simulink model "fu01"  (Simulink 5.0)
settings: Solver=ode45  StartTime=0.0  StopTime=inf  MaxStep=1/5000  MinStep=1/100000000  RelTol=1e-6
libraries: commcontsrc2 x1
settings Model: LastModifiedBy=efst

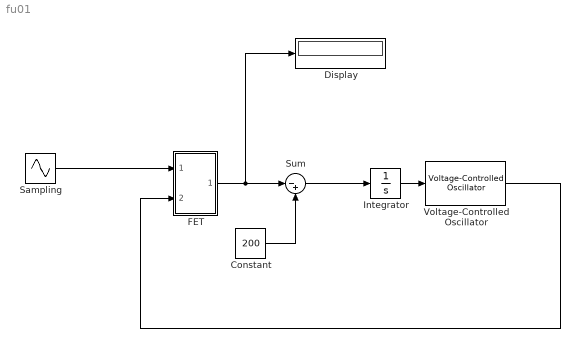
== system fu01 ==
  Constant : Constant  Value=200
  Display : Display
  FET : Subsystem
  Integrator : Integrator
  Sampling : Sin  Frequency=2*pi*1000  SampleTime=0
  Sum : Sum  Inputs=|-+  SaturateOnIntegerOverflow=on
  Voltage-Controlled Oscillator : commcontsrc2/Voltage-Controlled Oscillator  Ac=1  Fc=10  Kc=100  Ph=0
  wires:
  FET/1(Out1) -> Display/1, Sum/1
  Sampling/1 -> FET/1(In1)
  Integrator/1 -> Voltage-Controlled Oscillator/1
  Voltage-Controlled Oscillator/1 -> FET/2(In2)
  Sum/1 -> Integrator/1
  Constant/1 -> Sum/2

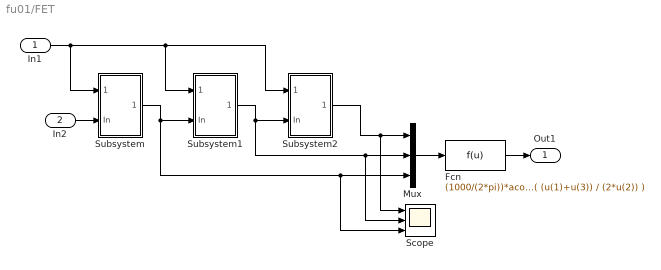
== system fu01/FET ==
  In1 : Inport
  In2 : Inport  Port=2
  Fcn : Fcn  Expr=(1000/(2*pi))*acos( (u(1)+u(3)) / (2*u(2)) )
  Mux : Mux  Inputs=3
  Scope : Scope  NumInputPorts=3
      settings: TimeRange=0.02  YMin=-1~-1~-1  YMax=1~1~1
  Subsystem : Subsystem
  Subsystem1 : Subsystem
  Subsystem2 : Subsystem
  Out1 : Outport
  wires:
  In1/1 -> Subsystem/1(Sample), Subsystem1/1(Sample), Subsystem2/1(Sample)
  Mux/1 -> Fcn/1
  Subsystem2/1(Out) -> Mux/1, Scope/1
  Subsystem1/1(Out) -> Subsystem2/2(In), Mux/2, Scope/2
  Subsystem/1(Out) -> Subsystem1/2(In), Mux/3, Scope/3
  In2/1 -> Subsystem/2(In)
  Fcn/1 -> Out1/1

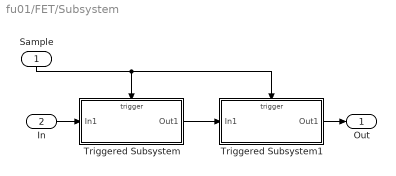
== system fu01/FET/Subsystem ==
  Sample : Inport  Orientation=down
  In : Inport  Port=2
  Triggered Subsystem : Subsystem  TreatAsAtomicUnit=on
  Triggered Subsystem1 : Subsystem  TreatAsAtomicUnit=on
  Out : Outport
  wires:
  Triggered Subsystem/1(Out1) -> Triggered Subsystem1/1(In1)
  Sample/1 -> Triggered Subsystem1/Trigger, Triggered Subsystem/Trigger
  In/1 -> Triggered Subsystem/1(In1)
  Triggered Subsystem1/1(Out1) -> Out/1

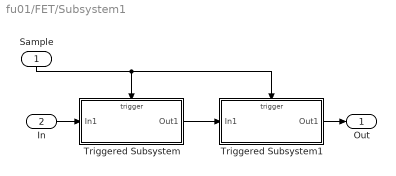
== system fu01/FET/Subsystem1 ==
  Sample : Inport  Orientation=down
  In : Inport  Port=2
  Triggered Subsystem : Subsystem  TreatAsAtomicUnit=on
  Triggered Subsystem1 : Subsystem  TreatAsAtomicUnit=on
  Out : Outport
  wires:
  Triggered Subsystem1/1(Out1) -> Out/1
  In/1 -> Triggered Subsystem/1(In1)
  Sample/1 -> Triggered Subsystem/Trigger, Triggered Subsystem1/Trigger
  Triggered Subsystem/1(Out1) -> Triggered Subsystem1/1(In1)

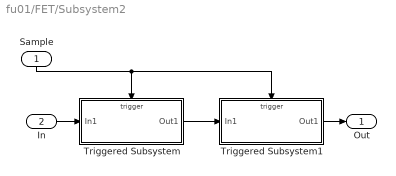
== system fu01/FET/Subsystem2 ==
  Sample : Inport  Orientation=down
  In : Inport  Port=2
  Triggered Subsystem : Subsystem  TreatAsAtomicUnit=on
  Triggered Subsystem1 : Subsystem  TreatAsAtomicUnit=on
  Out : Outport
  wires:
  Triggered Subsystem/1(Out1) -> Triggered Subsystem1/1(In1)
  Sample/1 -> Triggered Subsystem1/Trigger, Triggered Subsystem/Trigger
  In/1 -> Triggered Subsystem/1(In1)
  Triggered Subsystem1/1(Out1) -> Out/1

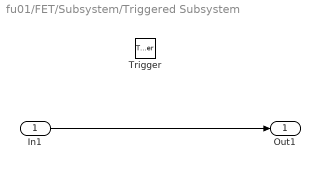
== system fu01/FET/Subsystem/Triggered Subsystem ==
  In1 : Inport
  Trigger : TriggerPort
  Out1 : Outport
  wires:
  In1/1 -> Out1/1

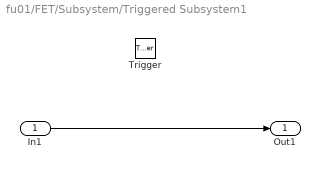
== system fu01/FET/Subsystem/Triggered Subsystem1 ==
  In1 : Inport
  Trigger : TriggerPort  TriggerType=falling
  Out1 : Outport
  wires:
  In1/1 -> Out1/1

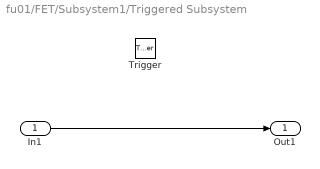
== system fu01/FET/Subsystem1/Triggered Subsystem ==
  In1 : Inport
  Trigger : TriggerPort
  Out1 : Outport
  wires:
  In1/1 -> Out1/1

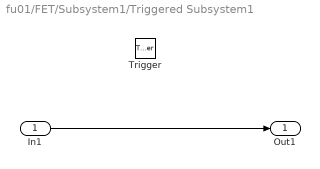
== system fu01/FET/Subsystem1/Triggered Subsystem1 ==
  In1 : Inport
  Trigger : TriggerPort  TriggerType=falling
  Out1 : Outport
  wires:
  In1/1 -> Out1/1

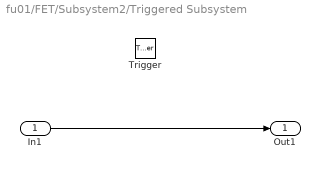
== system fu01/FET/Subsystem2/Triggered Subsystem ==
  In1 : Inport
  Trigger : TriggerPort
  Out1 : Outport
  wires:
  In1/1 -> Out1/1

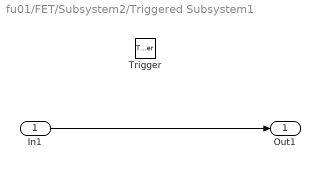
== system fu01/FET/Subsystem2/Triggered Subsystem1 ==
  In1 : Inport
  Trigger : TriggerPort  TriggerType=falling
  Out1 : Outport
  wires:
  In1/1 -> Out1/1
